simulink model "DifferentialEquation"  (R2020b)
settings: Solver=VariableStepAuto  StartTime=0.0  StopTime=10.0  RelTol=1e-3
settings Model: Creator=Training  LastModifiedBy=Training

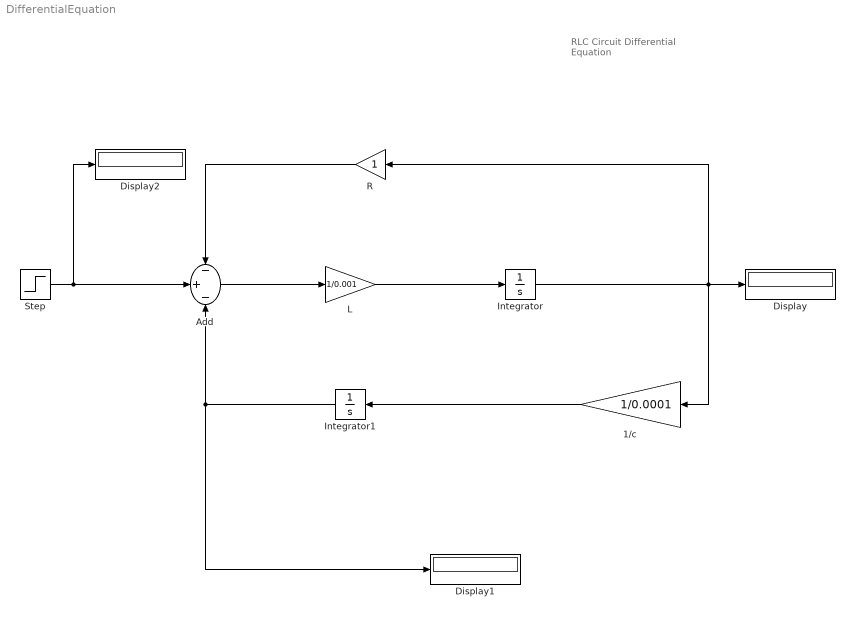
== system DifferentialEquation ==
  note: RLC Circuit
      | Differential Equation
  1/c : Gain  Gain=1/0.0001
  Add : Sum  Inputs=-+-
  Display : Display
  Display1 : Display
  Display2 : Display
  Integrator : Integrator
  Integrator1 : Integrator
  L : Gain  Gain=1/0.001
  R : Gain
  Step : Step  SampleTime=0
  wires:
  Step/1 -> Display2/1, Add/2
  R/1 -> Add/1
  Add/1 -> L/1
  L/1 -> Integrator/1
  Integrator/1 -> R/1, Display/1, 1/c/1
  Integrator1/1 -> Display1/1, Add/3
  1/c/1 -> Integrator1/1
